simulink model "Ex3_d_sim"  (R2021b)
settings: Solver=ode45  StartTime=0.0  StopTime=0.4  RelTol=1e-3  EnableMultiTasking=on
values from neighbouring files (symbols this model uses):
  D = 1e-5    (= 1e-05)    [Ex3_d.m]
  J = 1e-5    (= 1e-05)    [Ex3_d.m]
  K_e = 5e-2    (= 0.05)    [Ex3_d.m]
  K_t = 5e-2    (= 0.05)    [Ex3_d.m]
  L = 1e-3    (= 0.001)    [Ex3_d.m]
  R = 5.0    (= 5)    [Ex3_d.m]
  Td = 0.01    [Ex3_d.m]
settings Model: Creator=Shin  LastModifiedBy=mluser
settings SolverCC: AlgebraicLoopSolver=TrustRegion
settings DataIOCC: LimitDataPoints=on  SaveFormat=Array  ReturnWorkspaceOutputs=off
settings OptimizationCC: LifeSpan=inf
settings DebuggingCC: SolverPrmCheckMsg=warning  SFUnexpectedBacktrackingDiag=warning  SFNoUnconditionalDefaultTransitionDiag=warning  SFExecutionAtInitializationDiag=none  SFMachineParentedDataDiag=warning  ArithmeticOperatorsInVariantConditions=warning
settings HardwareCC: ProdBitPerPointer=32  ProdBitPerSizeT=32  ProdBitPerPtrDiffT=32  ProdLargestAtomicFloat=None  ProdIntDivRoundTo=Undefined  ProdEndianess=Unspecified  ProdWordSize=32  ProdHWDeviceType=32-bit Generic
settings ModelReferenceCC: PropagateSignalLabelsOutOfModel=off
settings SFSimCC: SimUseLocalCustomCode=off  CustomCodeUndefinedFunction=UseInterfaceOnly
settings RTWCC: RTWUseLocalCustomCode=off
settings CodeAppCC: StateflowObjectComments=on
settings GRTTargetCC: TargetLangStandard=C89/C90 (ANSI)
settings ConfigComp: CovMetricSettings=dw  CovSaveCumulativeToWorkspaceVar=on  CovSaveSingleToWorkspaceVar=on  CovExternalEMLEnable=off  CovSFcnEnable=off

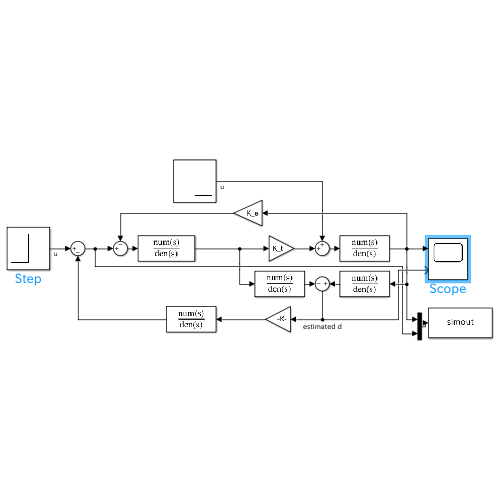
[thumbnail: Simulink's stored preview of the top-level diagram]
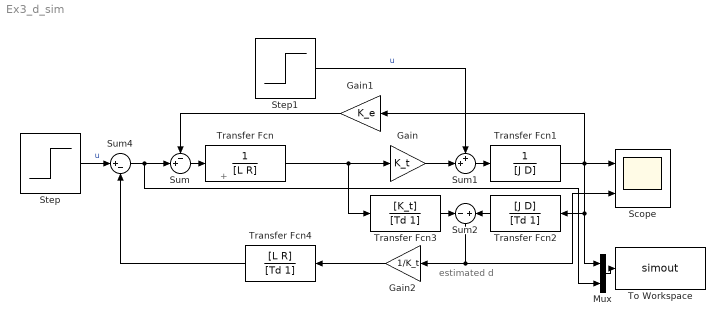
== system Ex3_d_sim ==
  note: estimated d
  note: +
  Gain : Gain  Gain=K_t
  Gain1 : Gain  Gain=K_e
  Gain2 : Gain  Gain=1/K_t
  Mux : Mux  Inputs=2
  Scope : Scope  NumInputPorts=2
  Step : Step  Time=0.01  SampleTime=0
  Step1 : Step  Time=0.15  After=-0.01  SampleTime=0
  Sum : Sum  Inputs=-+|
  Sum1 : Sum  Inputs=++|
  Sum2 : Sum  Inputs=-|+
  Sum4 : Sum  Inputs=|+-
  To Workspace : ToWorkspace  VariableName=simout  SaveFormat=Timeseries  SampleTime=-1
  Transfer Fcn : TransferFcn  Denominator=[L R]
  Transfer Fcn1 : TransferFcn  Denominator=[J D]
  Transfer Fcn2 : TransferFcn  Numerator=[J D]  Denominator=[Td 1]
  Transfer Fcn3 : TransferFcn  Numerator=[K_t]  Denominator=[Td 1]
  Transfer Fcn4 : TransferFcn  Numerator=[L R]  Denominator=[Td 1]
  wires:
  Mux/1 -> To Workspace/1
  Sum/1 -> Transfer Fcn/1
  Step1/1 -> Sum1/1  "u"
  Gain/1 -> Sum1/2
  Sum1/1 -> Transfer Fcn1/1
  Gain1/1 -> Sum/1
  Transfer Fcn1/1 -> Transfer Fcn2/1, Mux/1, Gain1/1, Scope/1
  Transfer Fcn3/1 -> Sum2/1
  Transfer Fcn/1 -> Transfer Fcn3/1, Gain/1
  Sum2/1 -> Scope/2, Gain2/1
  Transfer Fcn2/1 -> Sum2/2
  Sum4/1 -> Mux/2, Sum/2
  Step/1 -> Sum4/1  "u"
  Gain2/1 -> Transfer Fcn4/1
  Transfer Fcn4/1 -> Sum4/2
